simulink subsystem "RT_LeadLagDynamic_v1_0"  (R2025a)
settings: Solver=VariableStepAuto  StartTime=0.0  StopTime=100  RelTol=1e-3
undefined symbols (not defined in the file): RT_BEDistFrHingeLead_A, RT_BEDistFromEffSta_A, RT_BEMassFrHingeLead_A, RT_BladeLeadInertia_P, RT_HingeLeadPos_P, RT_RotorRadius_P
settings Model: DataDictionary=Rotor.sldd  EnableAccessToBaseWorkspace=off  DefaultTestHarness=LeadLagDynamic_Harness1  Creator=Admin  LastModifiedBy=Admin

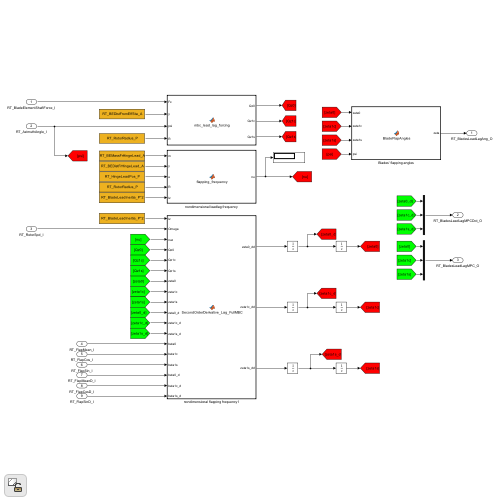
[thumbnail: Simulink's stored preview of the top-level diagram]
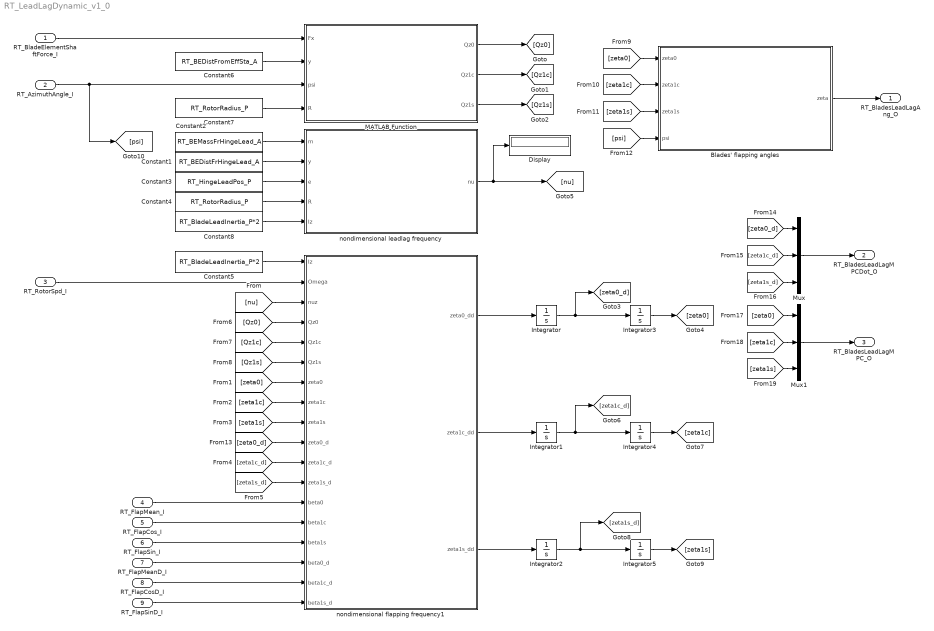
== system RT_LeadLagDynamic_v1_0 ==
  RT_BladeElementShaftForce_I : Inport
  RT_AzimuthAngle_I : Inport  Port=2
  RT_RotorSpd_I : Inport  Port=3
  RT_FlapMean_I : Inport  Port=4
  RT_FlapCos_I : Inport  Port=5
  RT_FlapSin_I : Inport  Port=6
  RT_FlapMeanD_I : Inport  Port=7
  RT_FlapCosD_I : Inport  Port=8
  RT_FlapSinD_I : Inport  Port=9
  Blades' flapping angles : MATLAB Function  TreatAsAtomicUnit=on
  Constant1 : Constant  Value=RT_BEDistFrHingeLead_A
  Constant2 : Constant  Value=RT_BEMassFrHingeLead_A
  Constant3 : Constant  Value=RT_HingeLeadPos_P
  Constant4 : Constant  Value=RT_RotorRadius_P
  Constant5 : Constant  Value=RT_BladeLeadInertia_P*2
  Constant6 : Constant  Value=RT_BEDistFromEffSta_A
  Constant7 : Constant  Value=RT_RotorRadius_P
  Constant8 : Constant  Value=RT_BladeLeadInertia_P*2
  Display : Display
  Integrator{,1..5} (6 alike) : Integrator
  MATLAB Function : MATLAB Function  TreatAsAtomicUnit=on
  Mux : Mux  Inputs=3
  Mux1 : Mux  Inputs=3
  nondimensional flapping frequency1 : MATLAB Function  TreatAsAtomicUnit=on
  nondimensional leadlag frequency : MATLAB Function  TreatAsAtomicUnit=on
  RT_BladesLeadLagAng_O : Outport
  RT_BladesLeadLagMPCDot_O : Outport  Port=2
  RT_BladesLeadLagMPC_O : Outport  Port=3
  wires:
  MATLAB Function/3(Qz1s) -> [Qz1s]
  Integrator1/1 -> Integrator4/1, [zeta1c_d]
  MATLAB Function/2(Qz1c) -> [Qz1c]
  Integrator5/1 -> [zeta1s]
  Integrator3/1 -> [zeta0]
  Constant1/1 -> nondimensional leadlag frequency/2(y)
  [zeta0] -> Blades' flapping angles/1(zeta0)
  nondimensional flapping frequency1/3(zeta1s_dd) -> Integrator2/1
  RT_BladeElementShaftForce_I/1 -> MATLAB Function/1(Fx)
  [psi] -> Blades' flapping angles/4(psi)
  Constant3/1 -> nondimensional leadlag frequency/3(e)
  Constant4/1 -> nondimensional leadlag frequency/4(R)
  Constant2/1 -> nondimensional leadlag frequency/1(m)
  nondimensional flapping frequency1/2(zeta1c_dd) -> Integrator1/1
  Integrator2/1 -> Integrator5/1, [zeta1s_d]
  Integrator/1 -> Integrator3/1, [zeta0_d]
  Constant6/1 -> MATLAB Function/2(y)
  nondimensional flapping frequency1/1(zeta0_dd) -> Integrator/1
  MATLAB Function/1(Qz0) -> [Qz0]
  Blades' flapping angles/1(zeta) -> RT_BladesLeadLagAng_O/1
  RT_AzimuthAngle_I/1 -> [psi], MATLAB Function/3(psi)
  [zeta1c] -> Blades' flapping angles/2(zeta1c)
  Integrator4/1 -> [zeta1c]
  [zeta1s] -> Blades' flapping angles/3(zeta1s)
  Constant8/1 -> nondimensional leadlag frequency/5(Iz)
  Constant7/1 -> MATLAB Function/4(R)
  Constant5/1 -> nondimensional flapping frequency1/1(Iz)
  RT_RotorSpd_I/1 -> nondimensional flapping frequency1/2(Omega)
  [nu] -> nondimensional flapping frequency1/3(nuz)
  [Qz0] -> nondimensional flapping frequency1/4(Qz0)
  [Qz1c] -> nondimensional flapping frequency1/5(Qz1c)
  [Qz1s] -> nondimensional flapping frequency1/6(Qz1s)
  [zeta0] -> nondimensional flapping frequency1/7(zeta0)
  [zeta1c] -> nondimensional flapping frequency1/8(zeta1c)
  [zeta1s] -> nondimensional flapping frequency1/9(zeta1s)
  [zeta1c_d] -> nondimensional flapping frequency1/11(zeta1c_d)
  RT_FlapMean_I/1 -> nondimensional flapping frequency1/13(beta0)
  RT_FlapCos_I/1 -> nondimensional flapping frequency1/14(beta1c)
  RT_FlapSin_I/1 -> nondimensional flapping frequency1/15(beta1s)
  RT_FlapCosD_I/1 -> nondimensional flapping frequency1/17(beta1c_d)
  RT_FlapSinD_I/1 -> nondimensional flapping frequency1/18(beta1s_d)
  RT_FlapMeanD_I/1 -> nondimensional flapping frequency1/16(beta0_d)
  [zeta1s_d] -> nondimensional flapping frequency1/12(zeta1s_d)
  [zeta0_d] -> nondimensional flapping frequency1/10(zeta0_d)
  nondimensional leadlag frequency/1(nu) -> Display/1, [nu]
  [zeta0_d] -> Mux/1
  [zeta1c_d] -> Mux/2
  [zeta1s_d] -> Mux/3
  Mux/1 -> RT_BladesLeadLagMPCDot_O/1
  [zeta1c] -> Mux1/2
  [zeta0] -> Mux1/1
  [zeta1s] -> Mux1/3
  Mux1/1 -> RT_BladesLeadLagMPC_O/1

== matlab function RT_LeadLagDynamic_v1_0/nondimensional leadlag frequency ==
  data: m input; nu output; y input; e input; R input; Iz input
function nu  = flapping_frequency(m, y, e, R, Iz)
% m   : [1 x Ns] radial element mass from hinge (kg)
% y   : [1 x Ns]  radial stations from hinge (m)  
% e   : [1 x 1]  hinge ratio with radius (-)
% R   : [1 x 1]  Radius of rotor blade
% Ib  :
% Returns blade flapping natural frequency (N·m)

      
    nu = e*R*m'*y/Iz;
end

== matlab function RT_LeadLagDynamic_v1_0/MATLAB Function ==
  data: Fx input; y input; psi input; Qz0 output; Qz1c output; Qz1s output; R input
function [Qz0, Qz1c, Qz1s] = mbc_lead_lag_forcing(Fx, y, psi, R)
% Extract MBC lag forcing from per-blade in-plane force array
% COMPILER SAFE VERSION FOR SIMULINK

    % 1. Đảm bảo biến đầu vào là vector cột
    psi = psi(:);
    y = y(:);
    
    % Lấy số lượng cánh (Nb) và số phân đoạn (Ns)
    Nb = length(psi); 
    Ns = length(y);   
    
    % 2. Khởi tạo kích thước cứng cho kết quả Moment
    Qz = zeros(Nb, 1);
    Fx_correct = zeros(Nb, Ns);
    
    % 3. LƯỚI LỌC COMPILER: Vượt rào bước giả lập kích thước [1x1]
    if numel(Fx) == (Nb * Ns)
        if size(Fx, 1) == Ns && size(Fx, 2) == Nb
            Fx_correct = Fx'; % Đảo từ [Ns x Nb] thành [Nb x Ns] nếu bị ngược
        elseif size(Fx, 1) == Nb && size(Fx, 2) == Ns
            Fx_correct = Fx;  % Chuẩn [Nb x Ns]
        else
            Fx_correct = reshape(Fx, [Nb, Ns]); % Ép mảng 1D thành [Nb x Ns]
        end
    else
        % Nếu Compiler đưa vào mảng 1x1, gán giá trị đó cho toàn bộ ô
        Fx_correct(:, :) = Fx(1); 
    end
    
    % 4. Tính Moment bằng vòng lặp để Compiler không bắt bẻ phép nhân ma trận
    for b = 1:Nb
        moment_sum = 0;
        for i = 1:Ns
            % Moment = Force * arm (với y là khoảng cách không thứ nguyên, nhân thêm R)
            moment_sum = moment_sum + Fx_correct(b, i) * y(i) * R;
        end
        Qz(b) = moment_sum; % Qz chắc chắn là [Nb x 1]
    end
    
    % 5. MBC extraction (Transform)
    Qz0  = sum(Qz) / Nb;
    Qz1c = (2 / Nb) * sum(Qz .* cos(psi));
    Qz1s = (2 / Nb) * sum(Qz .* sin(psi));
    
end

== matlab function RT_LeadLagDynamic_v1_0/nondimensional flapping frequency1 ==
  data: Iz input; Omega input; nuz input; Qz0 input; zeta0_dd output; Qz1c input; Qz1s input; zeta0 input; zeta1c input; zeta1s input; zeta0_d input; zeta1c_d input; zeta1s_d input; beta0 input; beta1c input; beta1s input; beta0_d input; beta1c_d input; beta1s_d input; zeta1c_dd output; zeta1s_dd output
function [zeta0_dd, zeta1c_dd, zeta1s_dd] = SecondOrderDerivative_Lag_FullMBC( ...
    Iz, Omega, nuz, ...
    Qz0, Qz1c, Qz1s, ...
    zeta0, zeta1c, zeta1s, ...
    zeta0_d, zeta1c_d, zeta1s_d, ...
    beta0, beta1c, beta1s, ...
    beta0_d, beta1c_d, beta1s_d)
% Full MBC lag dynamics — NO linearization of Coriolis term
%
% nuz = nu_zeta^2 (from leadlag_frequency)

    % ====== Coning lag ======
    % P0 = beta0*beta0_d + 0.5*beta1c*beta1c_d + 0.5*beta1s*beta1s_d
    P0 = beta0 * beta0_d ...
       + 0.5 * beta1c * beta1c_d ...
       + 0.5 * beta1s * beta1s_d;
    
    zeta0_dd = Qz0/Iz ...
             - nuz * Omega^2 * zeta0 ...
             - 2 * Omega * P0;
    
    % ====== Longitudinal cyclic lag ======
    % P1c = beta0*(beta1c_d + Omega*beta1s) + beta1c*beta0_d
    P1c = beta0 * beta1c_d ...
        + Omega * beta0 * beta1s ...
        + beta1c * beta0_d;
    
    zeta1c_dd = Qz1c/Iz ...
              - 2 * Omega * zeta1s_d ...
              - (nuz - 1) * Omega^2 * zeta1c ...
              - 2 * Omega * P1c;
    
    % ====== Lateral cyclic lag ======
    % P1s = beta0*(beta1s_d - Omega*beta1c) + beta1s*beta0_d
    P1s = beta0 * beta1s_d ...
        - Omega * beta0 * beta1c ...
        + beta1s * beta0_d;
    
    zeta1s_dd = Qz1s/Iz ...
              + 2 * Omega * zeta1c_d ...
              - (nuz - 1) * Omega^2 * zeta1s ...
              - 2 * Omega * P1s;
end

== matlab function RT_LeadLagDynamic_v1_0/Blades' flapping angles ==
  data: zeta0 input; zeta output; zeta1c input; zeta1s input; psi input
function zeta   = BladeFlapAngles(zeta0, zeta1c, zeta1s, psi)
    
    zeta = zeta0 + zeta1c*cos(psi) + zeta1s*sin(psi);
end
